simulink model "pfb_fir_generic_test_sim3"  (R2012b)
settings: Solver=VariableStepDiscrete  StartTime=0.0  StopTime=10.0  RelTol=1e-3
model workspace (MAT data in the model file):
  synci = [0 1 2 3 4 5 6 7 8 9 10 11 ... (589826 elements, 294913x2)]
  din0 = [0 1 2 3 4 5 6 7 8 9 10 11 ... (73730 elements, 36865x2)]
  din1 = [0 1 2 3 4 5 6 7 8 9 10 11 ... (73730 elements, 36865x2)]
  din2 = [0 1 2 3 4 5 6 7 8 9 10 11 ... (73730 elements, 36865x2)]
  din3 = [0 1 2 3 4 5 6 7 8 9 10 11 ... (73730 elements, 36865x2)]
  din4 = [0 1 2 3 4 5 6 7 8 9 10 11 ... (73730 elements, 36865x2)]
  din5 = [0 1 2 3 4 5 6 7 8 9 10 11 ... (73730 elements, 36865x2)]
  din6 = [0 1 2 3 4 5 6 7 8 9 10 11 ... (73730 elements, 36865x2)]
  din7 = [0 1 2 3 4 5 6 7 8 9 10 11 ... (73730 elements, 36865x2)]
libraries: xbsIndex_r4 x5585, casper_library_delays x1
(part 12 of 25)

== system pfb_fir_generic_test_sim3/pfb_fir_generic/pfb_fir_taps/bus_madd ==
  a : Inport
  b : Inport  Port=2
  c : Inport  Port=3
  en : Inport  Port=4
  Gateway Out{,1..23} (24 alike) : xbsIndex_r4/Gateway Out  inherit_from_input=off  hdl_port=on  timing_constraint=None  locs_specified=off  LOCs={}  UseAsDAC=off  DACChannel='1'  block_type=gatewayout
  To Workspace : ToWorkspace  VariableName=mult_ab_64  SampleTime=-1  SaveFormat=Timeseries
  To Workspace1 : ToWorkspace  VariableName=mult_ab_c_64  SampleTime=-1  SaveFormat=Timeseries
  To Workspace10 : ToWorkspace  VariableName=mult_a33  SampleTime=-1  SaveFormat=Structure With Time
  To Workspace11 : ToWorkspace  VariableName=mult_a32  SampleTime=-1  SaveFormat=Structure With Time
  To Workspace12 : ToWorkspace  VariableName=mult_a31  SampleTime=-1  SaveFormat=Structure With Time
  To Workspace13 : ToWorkspace  VariableName=mult_b33  SampleTime=-1  SaveFormat=Structure With Time
  To Workspace14 : ToWorkspace  VariableName=mult_b32  SampleTime=-1  SaveFormat=Structure With Time
  To Workspace15 : ToWorkspace  VariableName=mult_b31  SampleTime=-1  SaveFormat=Structure With Time
  To Workspace16 : ToWorkspace  VariableName=add_b_32  SampleTime=-1  SaveFormat=Structure With Time
  To Workspace17 : ToWorkspace  VariableName=add_b_33  SampleTime=-1  SaveFormat=Structure With Time
  To Workspace18 : ToWorkspace  VariableName=add_b_16  SampleTime=-1  SaveFormat=Structure With Time
  To Workspace19 : ToWorkspace  VariableName=add_b_48  SampleTime=-1  SaveFormat=Structure With Time
  To Workspace2 : ToWorkspace  VariableName=mult_ab_32  SampleTime=-1  SaveFormat=Structure With Time
  To Workspace20 : ToWorkspace  VariableName=add_b_17  SampleTime=-1  SaveFormat=Structure With Time
  To Workspace21 : ToWorkspace  VariableName=add_b_15  SampleTime=-1  SaveFormat=Structure With Time
  To Workspace22 : ToWorkspace  VariableName=add_b_47  SampleTime=-1  SaveFormat=Structure With Time
  To Workspace23 : ToWorkspace  VariableName=add_b_49  SampleTime=-1  SaveFormat=Structure With Time
  To Workspace3 : ToWorkspace  VariableName=mult_ab_c_33  SampleTime=-1  SaveFormat=Structure With Time
  To Workspace4 : ToWorkspace  VariableName=mult_ab_c_31  SampleTime=-1  SaveFormat=Structure With Time
  To Workspace5 : ToWorkspace  VariableName=mult_ab_33  SampleTime=-1  SaveFormat=Structure With Time
  To Workspace6 : ToWorkspace  VariableName=mult_ab_31  SampleTime=-1  SaveFormat=Structure With Time
  To Workspace7 : ToWorkspace  VariableName=mult_ab_c32  SampleTime=-1  SaveFormat=Structure With Time
  To Workspace8 : ToWorkspace  VariableName=mult_ab_c_34  SampleTime=-1  SaveFormat=Structure With Time
  To Workspace9 : ToWorkspace  VariableName=add_b_34  SampleTime=-1  SaveFormat=Structure With Time
  a*b+c_bussify : Subsystem  AncestorBlock=casper_library_flow_control/bus_create  mask(bus_create){inputNum=64}
      mask prompts: inputNum "Number of inputs:"
      mask init:
      | bus_create_init(gcb,...
      |     'inputNum', inputNum);
  a_debus : Subsystem  AncestorBlock=casper_library_flow_control/bus_expand  mask(bus_expand){mode=divisions of arbitrary size, outputNum=1, outputWidth=[10 10 10 10 10 10 10 10 10 10 10 10 10 10 10 10 10 10 10 10 10 10 10 10 10 10 10 10 10 10 10 10 10 10 10 10 10 10 10 10 10 10 10 10 10 10 10 10 10 10 10 10 10 10 10 10 10 10 10 10 10 10 10 10], outputBinaryPt=[9 9 9 9 9 9 9 9 9 9 9 9 9 9 9 9 9 9 9 9 9 9 9 9 9 9 9 9 9 9 9 9 9 9 9 9 9 9 9 9 9 9 9 9 9 9 9 9 9 9 9 9 9 9 9 9 9 9 9 9 9 9 9 9], outputArithmeticType=[1 1 1 1 1 1 1 1 1 1 1 1 1 1 1 1 1 1 1 1 1 1 1 1 1 1 1 1 1 1 1 1 1 1 1 1 1 1 1 1 1 1 1 1 1 1 1 1 1 1 1 1 1 1 1 1 1 1 1 1 1 1 1 1], show_format=on, outputToWorkspace=on, variablePrefix=mult_a, outputToModelAsWell=on}
      mask prompts: outputNum "Number of outputs:"; outputWidth "Output width [msb ... lsb]:"; outputBinaryPt "Output binary point position [msb ... lsb]:"; outputArithmeticType "Output arithmetic type (ufix=0, fix=1, bool=2) [msb ... lsb]:"; show_format "Print format string?"; outputToWorkspace "Output to workspace?"; variablePrefix "Variable name prefix:"; outputToModelAsWell "Output to model as well?"
      mask help:
      | Expands a 'bus' made using a bus_create or Xilinx
      | concat block.
      | The input will be divided into the specified number
      | of outputs with the specified arithmetic types.
      | Divisions are made from most significant bit.
      mask init: same as pfb_fir_generic_test_sim3/pfb_fir_generic/bus_expand
      settings: AttributesFormatString=64 outputs: f10.9,f10.9,f10.9,f10.9,f10.9,f10.9,f10.9,f10.9,f10.9,f10.9,f10.9,f10.9,f10.9,f10.9,f10.9,f10.9,f10.9,f10.9,f10.9,f10.9,f10.9,f10.9,f10.9,f10.9,f10.9,f10.9,f10.9,f10.9,f10.9,f10.9,f10.9,f10.9,f10.9,f10.9,f10.9,f10.9,f10.9,f10.9,f10.9,f10.9,f10.9,f10.9,f10.9,f10.9,f10.9,f10.9,f10.9,f10.9,f10.9,f10.9,f10.9,f10.9,f10.9,f10.9,f10.9,f10.9,f10.9,f10.9,f10.9,f10.9,f10.9,f10.9,f10.9,f10.9,, mult_a_?
      mask TypeOptions mode: divisions of equal size | divisions of arbitrary size
      mask Callback mode: bus_expand_callback();
      mask Callback outputWidth: bus_expand_callback();
      mask Callback outputToWorkspace: bus_expand_callback();
  addsub{1..16} (16 alike) : xbsIndex_r4/AddSub  mode=Addition  use_carryin=off  use_carryout=off  en=on  latency=1  precision=User Defined  arith_type="Signed  (2's comp)"  n_bits=28  bin_pt=26  quantization=Truncate  overflow=Wrap  dbl_ovrd=off  use_behavioral_HDL=on  hw_selection=Fabric  pipelined=on  block_type=addsub
  addsub{17..32} (16 alike) : xbsIndex_r4/AddSub  mode=Addition  use_carryin=off  use_carryout=off  en=on  latency=1  precision=User Defined  arith_type="Signed  (2's comp)"  n_bits=29  bin_pt=26  quantization=Truncate  overflow=Wrap  dbl_ovrd=off  use_behavioral_HDL=on  hw_selection=Fabric  pipelined=on  block_type=addsub
  addsub{33..48} (16 alike) : xbsIndex_r4/AddSub  mode=Addition  use_carryin=off  use_carryout=off  en=on  latency=1  precision=User Defined  arith_type="Signed  (2's comp)"  n_bits=30  bin_pt=26  quantization=Truncate  overflow=Wrap  dbl_ovrd=off  use_behavioral_HDL=on  hw_selection=Fabric  pipelined=on  block_type=addsub
  addsub{49..64} (16 alike) : xbsIndex_r4/AddSub  mode=Addition  use_carryin=off  use_carryout=off  en=on  latency=1  precision=User Defined  arith_type="Signed  (2's comp)"  n_bits=31  bin_pt=26  quantization=Truncate  overflow=Wrap  dbl_ovrd=off  use_behavioral_HDL=on  hw_selection=Fabric  pipelined=on  block_type=addsub
  b_debus : Subsystem  AncestorBlock=casper_library_flow_control/bus_expand  mask(bus_expand){mode=divisions of arbitrary size, outputNum=1, outputWidth=[18 18 18 18 18 18 18 18 18 18 18 18 18 18 18 18 18 18 18 18 18 18 18 18 18 18 18 18 18 18 18 18 18 18 18 18 18 18 18 18 18 18 18 18 18 18 18 18 18 18 18 18 18 18 18 18 18 18 18 18 18 18 18 18], outputBinaryPt=[17 17 17 17 17 17 17 17 17 17 17 17 17 17 17 17 17 17 17 17 17 17 17 17 17 17 17 17 17 17 17 17 17 17 17 17 17 17 17 17 17 17 17 17 17 17 17 17 17 17 17 17 17 17 17 17 17 17 17 17 17 17 17 17], outputArithmeticType=[1 1 1 1 1 1 1 1 1 1 1 1 1 1 1 1 1 1 1 1 1 1 1 1 1 1 1 1 1 1 1 1 1 1 1 1 1 1 1 1 1 1 1 1 1 1 1 1 1 1 1 1 1 1 1 1 1 1 1 1 1 1 1 1], show_format=on, outputToWorkspace=on, variablePrefix=mult_b, outputToModelAsWell=on}
      mask prompts: outputNum "Number of outputs:"; outputWidth "Output width [msb ... lsb]:"; outputBinaryPt "Output binary point position [msb ... lsb]:"; outputArithmeticType "Output arithmetic type (ufix=0, fix=1, bool=2) [msb ... lsb]:"; show_format "Print format string?"; outputToWorkspace "Output to workspace?"; variablePrefix "Variable name prefix:"; outputToModelAsWell "Output to model as well?"
      mask help:
      | Expands a 'bus' made using a bus_create or Xilinx
      | concat block.
      | The input will be divided into the specified number
      | of outputs with the specified arithmetic types.
      | Divisions are made from most significant bit.
      mask init: same as pfb_fir_generic_test_sim3/pfb_fir_generic/bus_expand
      settings: AttributesFormatString=64 outputs: f18.17,f18.17,f18.17,f18.17,f18.17,f18.17,f18.17,f18.17,f18.17,f18.17,f18.17,f18.17,f18.17,f18.17,f18.17,f18.17,f18.17,f18.17,f18.17,f18.17,f18.17,f18.17,f18.17,f18.17,f18.17,f18.17,f18.17,f18.17,f18.17,f18.17,f18.17,f18.17,f18.17,f18.17,f18.17,f18.17,f18.17,f18.17,f18.17,f18.17,f18.17,f18.17,f18.17,f18.17,f18.17,f18.17,f18.17,f18.17,f18.17,f18.17,f18.17,f18.17,f18.17,f18.17,f18.17,f18.17,f18.17,f18.17,f18.17,f18.17,f18.17,f18.17,f18.17,f18.17,, mult_b_?
      mask TypeOptions mode: divisions of equal size | divisions of arbitrary size
      mask Callback mode: bus_expand_callback();
      mask Callback outputWidth: bus_expand_callback();
      mask Callback outputToWorkspace: bus_expand_callback();
  c_debus : Subsystem  AncestorBlock=casper_library_flow_control/bus_expand  mask(bus_expand){mode=divisions of arbitrary size, outputNum=1, outputWidth=[28 28 28 28 28 28 28 28 28 28 28 28 28 28 28 28 28 28 28 28 28 28 28 28 28 28 28 28 28 28 28 28 29 29 29 29 29 29 29 29 29 29 29 29 29 29 29 29 30 30 30 30 30 30 30 30 30 30 30 30 30 30 30 30], outputBinaryPt=[26 26 26 26 26 26 26 26 26 26 26 26 26 26 26 26 26 26 26 26 26 26 26 26 26 26 26 26 26 26 26 26 26 26 26 26 26 26 26 26 26 26 26 26 26 26 26 26 26 26 26 26 26 26 26 26 26 26 26 26 26 26 26 26], outputArithmeticType=[1 1 1 1 1 1 1 1 1 1 1 1 1 1 1 1 1 1 1 1 1 1 1 1 1 1 1 1 1 1 1 1 1 1 1 1 1 1 1 1 1 1 1 1 1 1 1 1 1 1 1 1 1 1 1 1 1 1 1 1 1 1 1 1], show_format=on, outputToWorkspace=on, variablePrefix=add_c, outputToModelAsWell=on}
      mask prompts: outputNum "Number of outputs:"; outputWidth "Output width [msb ... lsb]:"; outputBinaryPt "Output binary point position [msb ... lsb]:"; outputArithmeticType "Output arithmetic type (ufix=0, fix=1, bool=2) [msb ... lsb]:"; show_format "Print format string?"; outputToWorkspace "Output to workspace?"; variablePrefix "Variable name prefix:"; outputToModelAsWell "Output to model as well?"
      mask help:
      | Expands a 'bus' made using a bus_create or Xilinx
      | concat block.
      | The input will be divided into the specified number
      | of outputs with the specified arithmetic types.
      | Divisions are made from most significant bit.
      mask init: same as pfb_fir_generic_test_sim3/pfb_fir_generic/bus_expand
      settings: AttributesFormatString=64 outputs: f28.26,f28.26,f28.26,f28.26,f28.26,f28.26,f28.26,f28.26,f28.26,f28.26,f28.26,f28.26,f28.26,f28.26,f28.26,f28.26,f28.26,f28.26,f28.26,f28.26,f28.26,f28.26,f28.26,f28.26,f28.26,f28.26,f28.26,f28.26,f28.26,f28.26,f28.26,f28.26,f29.26,f29.26,f29.26,f29.26,f29.26,f29.26,f29.26,f29.26,f29.26,f29.26,f29.26,f29.26,f29.26,f29.26,f29.26,f29.26,f30.26,f30.26,f30.26,f30.26,f30.26,f30.26,f30.26,f30.26,f30.26,f30.26,f30.26,f30.26,f30.26,f30.26,f30.26,f30.26,, add_c_?
      mask TypeOptions mode: divisions of equal size | divisions of arbitrary size
      mask Callback mode: bus_expand_callback();
      mask Callback outputWidth: bus_expand_callback();
      mask Callback outputToWorkspace: bus_expand_callback();
  den0 : xbsIndex_r4/Delay  rst=off  infoeditControl=Selection of Reset will increase slice count due to use of real FFs and instead of SRLs  en=off  latency=3  dbl_ovrd=off  reg_retiming=on  block_type=delay
  den1 : xbsIndex_r4/Delay  rst=off  infoeditControl=Selection of Reset will increase slice count due to use of real FFs and instead of SRLs  en=off  latency=1  dbl_ovrd=off  reg_retiming=on  block_type=delay
  den2 : xbsIndex_r4/Delay  rst=off  infoeditControl=Selection of Reset will increase slice count due to use of real FFs and instead of SRLs  en=off  latency=1  dbl_ovrd=off  reg_retiming=on  block_type=delay
  en_debus1 : Subsystem  AncestorBlock=casper_library_flow_control/bus_expand  mask(bus_expand){mode=divisions of equal size, outputNum=64, outputWidth=1, outputBinaryPt=0, outputArithmeticType=2, show_format=on, outputToWorkspace=on, variablePrefix=add_en, outputToModelAsWell=on}
      mask prompts: outputNum "Number of outputs:"; outputWidth "Output width:"; outputBinaryPt "Output binary point position:"; outputArithmeticType "Output arithmetic type (ufix=0, fix=1, bool=2):"; show_format "Print format string?"; outputToWorkspace "Output to workspace?"; variablePrefix "Variable name prefix:"; outputToModelAsWell "Output to model as well?"
      mask help:
      | Expands a 'bus' made using a bus_create or Xilinx
      | concat block.
      | The input will be divided into the specified number
      | of outputs with the specified arithmetic types.
      | Divisions are made from most significant bit.
      mask init: same as pfb_fir_generic_test_sim3/pfb_fir_generic/bus_expand
      settings: AttributesFormatString=64 outputs: b,b,b,b,b,b,b,b,b,b,b,b,b,b,b,b,b,b,b,b,b,b,b,b,b,b,b,b,b,b,b,b,b,b,b,b,b,b,b,b,b,b,b,b,b,b,b,b,b,b,b,b,b,b,b,b,b,b,b,b,b,b,b,b,, add_en_?
      mask TypeOptions mode: divisions of equal size | divisions of arbitrary size
      mask Callback mode: bus_expand_callback();
      mask Callback outputWidth: bus_expand_callback();
      mask Callback outputToWorkspace: bus_expand_callback();
  mult{1..64} (64 alike) : xbsIndex_r4/Mult  precision=Full  arith_type="Signed  (2's comp)"  n_bits=16  bin_pt=14  quantization=Truncate  overflow=Wrap  en=off  latency=3  dbl_ovrd=off  use_behavioral_HDL=on  opt=Speed  use_embedded=off  optimum_pipeline=off  pipeline=on  use_rpm=on  placement_style=Triangular  block_type=mult
  repa : Subsystem  AncestorBlock=casper_library_bus/bus_replicate  mask(bus_replicate){replication=1, latency=1, misc=off, implementation=core}
      mask prompts: replication "replication factor"; misc "misc support"; implementation "delay implementation"
      mask help: Output bus formed by replicating input bus a number of times
      mask init:
      | bus_replicate_init(gcb, ...
      |     'replication', replication, ...
      |     'latency', latency, ...
      |     'implementation', implementation, ...
      |     'misc', misc);
      mask TypeOptions implementation: core | behavioral
  repb : Subsystem  AncestorBlock=casper_library_bus/bus_replicate  mask(bus_replicate){replication=1, latency=1, misc=off, implementation=core}
      mask prompts: replication "replication factor"; misc "misc support"; implementation "delay implementation"
      mask help: Output bus formed by replicating input bus a number of times
      mask init:
      | bus_replicate_init(gcb, ...
      |     'replication', replication, ...
      |     'latency', latency, ...
      |     'implementation', implementation, ...
      |     'misc', misc);
      mask TypeOptions implementation: core | behavioral
  repen1 : Subsystem  AncestorBlock=casper_library_bus/bus_replicate  mask(bus_replicate){replication=64, latency=2, misc=off, implementation=core}
      mask prompts: replication "replication factor"; misc "misc support"; implementation "delay implementation"
      mask help: Output bus formed by replicating input bus a number of times
      mask init:
      | bus_replicate_init(gcb, ...
      |     'replication', replication, ...
      |     'latency', latency, ...
      |     'implementation', implementation, ...
      |     'misc', misc);
      mask TypeOptions implementation: core | behavioral
  a*b+c : Outport
  dvalid : Outport  Port=2
  wires:
  a/1 -> repa/1(in)
  b/1 -> repb/1(in)
  repa/1(out) -> a_debus/1(bus_in)
  repb/1(out) -> b_debus/1(bus_in)
  a_debus/1(msb_out64) -> mult1/1
  b_debus/1(msb_out64) -> mult1/2
  a_debus/2(out63) -> mult2/1
  b_debus/2(out63) -> mult2/2
  a_debus/3(out62) -> mult3/1
  b_debus/3(out62) -> mult3/2
  a_debus/4(out61) -> mult4/1
  b_debus/4(out61) -> mult4/2
  a_debus/5(out60) -> mult5/1
  b_debus/5(out60) -> mult5/2
  a_debus/6(out59) -> mult6/1
  b_debus/6(out59) -> mult6/2
  a_debus/7(out58) -> mult7/1
  b_debus/7(out58) -> mult7/2
  a_debus/8(out57) -> mult8/1
  b_debus/8(out57) -> mult8/2
  a_debus/9(out56) -> mult9/1
  b_debus/9(out56) -> mult9/2
  a_debus/10(out55) -> mult10/1
  b_debus/10(out55) -> mult10/2
  a_debus/11(out54) -> mult11/1
  b_debus/11(out54) -> mult11/2
  a_debus/12(out53) -> mult12/1
  b_debus/12(out53) -> mult12/2
  a_debus/13(out52) -> mult13/1
  b_debus/13(out52) -> mult13/2
  a_debus/14(out51) -> mult14/1
  b_debus/14(out51) -> mult14/2
  a_debus/15(out50) -> mult15/1
  b_debus/15(out50) -> mult15/2
  a_debus/16(out49) -> mult16/1
  b_debus/16(out49) -> mult16/2
  a_debus/17(out48) -> mult17/1
  b_debus/17(out48) -> mult17/2
  a_debus/18(out47) -> mult18/1
  b_debus/18(out47) -> mult18/2
  a_debus/19(out46) -> mult19/1
  b_debus/19(out46) -> mult19/2
  a_debus/20(out45) -> mult20/1
  b_debus/20(out45) -> mult20/2
  a_debus/21(out44) -> mult21/1
  b_debus/21(out44) -> mult21/2
  a_debus/22(out43) -> mult22/1
  b_debus/22(out43) -> mult22/2
  a_debus/23(out42) -> mult23/1
  b_debus/23(out42) -> mult23/2
  a_debus/24(out41) -> mult24/1
  b_debus/24(out41) -> mult24/2
  a_debus/25(out40) -> mult25/1
  b_debus/25(out40) -> mult25/2
  a_debus/26(out39) -> mult26/1
  b_debus/26(out39) -> mult26/2
  a_debus/27(out38) -> mult27/1
  b_debus/27(out38) -> mult27/2
  a_debus/28(out37) -> mult28/1
  b_debus/28(out37) -> mult28/2
  a_debus/29(out36) -> mult29/1
  b_debus/29(out36) -> mult29/2
  a_debus/30(out35) -> mult30/1
  b_debus/30(out35) -> mult30/2
  a_debus/31(out34) -> mult31/1
  b_debus/31(out34) -> mult31/2
  a_debus/32(out33) -> Gateway Out10/1, mult32/1
  b_debus/32(out33) -> Gateway Out13/1, mult32/2
  a_debus/33(out32) -> Gateway Out11/1, mult33/1
  b_debus/33(out32) -> Gateway Out14/1, mult33/2
  a_debus/34(out31) -> Gateway Out12/1, mult34/1
  b_debus/34(out31) -> Gateway Out15/1, mult34/2
  a_debus/35(out30) -> mult35/1
  b_debus/35(out30) -> mult35/2
  a_debus/36(out29) -> mult36/1
  b_debus/36(out29) -> mult36/2
  a_debus/37(out28) -> mult37/1
  b_debus/37(out28) -> mult37/2
  a_debus/38(out27) -> mult38/1
  b_debus/38(out27) -> mult38/2
  a_debus/39(out26) -> mult39/1
  b_debus/39(out26) -> mult39/2
  a_debus/40(out25) -> mult40/1
  b_debus/40(out25) -> mult40/2
  a_debus/41(out24) -> mult41/1
  b_debus/41(out24) -> mult41/2
  a_debus/42(out23) -> mult42/1
  b_debus/42(out23) -> mult42/2
  a_debus/43(out22) -> mult43/1
  b_debus/43(out22) -> mult43/2
  a_debus/44(out21) -> mult44/1
  b_debus/44(out21) -> mult44/2
  a_debus/45(out20) -> mult45/1
  b_debus/45(out20) -> mult45/2
  a_debus/46(out19) -> mult46/1
  b_debus/46(out19) -> mult46/2
  a_debus/47(out18) -> mult47/1
  b_debus/47(out18) -> mult47/2
  a_debus/48(out17) -> mult48/1
  b_debus/48(out17) -> mult48/2
  a_debus/49(out16) -> mult49/1
  b_debus/49(out16) -> mult49/2
  a_debus/50(out15) -> mult50/1
  b_debus/50(out15) -> mult50/2
  a_debus/51(out14) -> mult51/1
  b_debus/51(out14) -> mult51/2
  a_debus/52(out13) -> mult52/1
  b_debus/52(out13) -> mult52/2
  a_debus/53(out12) -> mult53/1
  b_debus/53(out12) -> mult53/2
  a_debus/54(out11) -> mult54/1
  b_debus/54(out11) -> mult54/2
  a_debus/55(out10) -> mult55/1
  b_debus/55(out10) -> mult55/2
  a_debus/56(out9) -> mult56/1
  b_debus/56(out9) -> mult56/2
  a_debus/57(out8) -> mult57/1
  b_debus/57(out8) -> mult57/2
  a_debus/58(out7) -> mult58/1
  b_debus/58(out7) -> mult58/2
  a_debus/59(out6) -> mult59/1
  b_debus/59(out6) -> mult59/2
  a_debus/60(out5) -> mult60/1
  b_debus/60(out5) -> mult60/2
  a_debus/61(out4) -> mult61/1
  b_debus/61(out4) -> mult61/2
  a_debus/62(out3) -> mult62/1
  b_debus/62(out3) -> mult62/2
  a_debus/63(out2) -> mult63/1
  b_debus/63(out2) -> mult63/2
  a_debus/64(lsb_out1) -> mult64/1
  b_debus/64(lsb_out1) -> mult64/2
  en/1 -> den0/1, repen1/1(in)
  den0/1 -> den1/1
  c/1 -> c_debus/1(bus_in)
  repen1/1(out) -> en_debus1/1(bus_in)
  mult1/1 -> Gateway Out/1, addsub1/1
  c_debus/1(msb_out64) -> addsub1/2
  en_debus1/1(msb_out64) -> addsub1/3
  mult2/1 -> addsub2/1
  c_debus/2(out63) -> addsub2/2
  en_debus1/2(out63) -> addsub2/3
  mult3/1 -> addsub3/1
  c_debus/3(out62) -> addsub3/2
  en_debus1/3(out62) -> addsub3/3
  mult4/1 -> addsub4/1
  c_debus/4(out61) -> addsub4/2
  en_debus1/4(out61) -> addsub4/3
  mult5/1 -> addsub5/1
  c_debus/5(out60) -> addsub5/2
  en_debus1/5(out60) -> addsub5/3
  mult6/1 -> addsub6/1
  c_debus/6(out59) -> addsub6/2
  en_debus1/6(out59) -> addsub6/3
  mult7/1 -> addsub7/1
  c_debus/7(out58) -> addsub7/2
  en_debus1/7(out58) -> addsub7/3
  mult8/1 -> addsub8/1
  c_debus/8(out57) -> addsub8/2
  en_debus1/8(out57) -> addsub8/3
  mult9/1 -> addsub9/1
  c_debus/9(out56) -> addsub9/2
  en_debus1/9(out56) -> addsub9/3
  mult10/1 -> addsub10/1
  c_debus/10(out55) -> addsub10/2
  en_debus1/10(out55) -> addsub10/3
  mult11/1 -> addsub11/1
  c_debus/11(out54) -> addsub11/2
  en_debus1/11(out54) -> addsub11/3
  mult12/1 -> addsub12/1
  c_debus/12(out53) -> addsub12/2
  en_debus1/12(out53) -> addsub12/3
  mult13/1 -> addsub13/1
  c_debus/13(out52) -> addsub13/2
  en_debus1/13(out52) -> addsub13/3
  mult14/1 -> addsub14/1
  c_debus/14(out51) -> addsub14/2
  en_debus1/14(out51) -> addsub14/3
  mult15/1 -> addsub15/1
  c_debus/15(out50) -> Gateway Out21/1, addsub15/2
  en_debus1/15(out50) -> addsub15/3
  mult16/1 -> addsub16/1
  c_debus/16(out49) -> Gateway Out18/1, addsub16/2
  en_debus1/16(out49) -> addsub16/3
  mult17/1 -> addsub17/1
  c_debus/17(out48) -> Gateway Out20/1, addsub17/2
  en_debus1/17(out48) -> addsub17/3
  mult18/1 -> addsub18/1
  c_debus/18(out47) -> addsub18/2
  en_debus1/18(out47) -> addsub18/3
  mult19/1 -> addsub19/1
  c_debus/19(out46) -> addsub19/2
  en_debus1/19(out46) -> addsub19/3
  mult20/1 -> addsub20/1
  c_debus/20(out45) -> addsub20/2
  en_debus1/20(out45) -> addsub20/3
  mult21/1 -> addsub21/1
  c_debus/21(out44) -> addsub21/2
  en_debus1/21(out44) -> addsub21/3
  mult22/1 -> addsub22/1
  c_debus/22(out43) -> addsub22/2
  en_debus1/22(out43) -> addsub22/3
  mult23/1 -> addsub23/1
  c_debus/23(out42) -> addsub23/2
  en_debus1/23(out42) -> addsub23/3
  mult24/1 -> addsub24/1
  c_debus/24(out41) -> addsub24/2
  en_debus1/24(out41) -> addsub24/3
  mult25/1 -> addsub25/1
  c_debus/25(out40) -> addsub25/2
  en_debus1/25(out40) -> addsub25/3
  mult26/1 -> addsub26/1
  c_debus/26(out39) -> addsub26/2
  en_debus1/26(out39) -> addsub26/3
  mult27/1 -> addsub27/1
  c_debus/27(out38) -> addsub27/2
  en_debus1/27(out38) -> addsub27/3
  mult28/1 -> addsub28/1
  c_debus/28(out37) -> addsub28/2
  en_debus1/28(out37) -> addsub28/3
  mult29/1 -> addsub29/1
  c_debus/29(out36) -> addsub29/2
  en_debus1/29(out36) -> addsub29/3
  mult30/1 -> addsub30/1
  c_debus/30(out35) -> addsub30/2
  en_debus1/30(out35) -> addsub30/3
  mult31/1 -> addsub31/1
  c_debus/31(out34) -> addsub31/2
  en_debus1/31(out34) -> addsub31/3
  mult32/1 -> Gateway Out5/1, addsub32/1
  c_debus/32(out33) -> Gateway Out16/1, addsub32/2
  en_debus1/32(out33) -> addsub32/3
  mult33/1 -> Gateway Out2/1, addsub33/1
  en_debus1/33(out32) -> addsub33/3
  mult34/1 -> Gateway Out6/1, addsub34/1
  c_debus/34(out31) -> Gateway Out17/1, addsub34/2
  en_debus1/34(out31) -> addsub34/3
  mult35/1 -> addsub35/1
  c_debus/35(out30) -> addsub35/2
  en_debus1/35(out30) -> addsub35/3
  mult36/1 -> addsub36/1
  c_debus/36(out29) -> addsub36/2
  en_debus1/36(out29) -> addsub36/3
  mult37/1 -> addsub37/1
  c_debus/37(out28) -> addsub37/2
  en_debus1/37(out28) -> addsub37/3
  mult38/1 -> addsub38/1
  c_debus/38(out27) -> addsub38/2
  en_debus1/38(out27) -> addsub38/3
  mult39/1 -> addsub39/1
  c_debus/39(out26) -> addsub39/2
  en_debus1/39(out26) -> addsub39/3
  mult40/1 -> addsub40/1
  c_debus/40(out25) -> addsub40/2
  en_debus1/40(out25) -> addsub40/3
  mult41/1 -> addsub41/1
  c_debus/41(out24) -> addsub41/2
  en_debus1/41(out24) -> addsub41/3
  mult42/1 -> addsub42/1
  c_debus/42(out23) -> addsub42/2
  en_debus1/42(out23) -> addsub42/3
  mult43/1 -> addsub43/1
  c_debus/43(out22) -> addsub43/2
  en_debus1/43(out22) -> addsub43/3
  mult44/1 -> addsub44/1
  c_debus/44(out21) -> addsub44/2
  en_debus1/44(out21) -> addsub44/3
  mult45/1 -> addsub45/1
  c_debus/45(out20) -> addsub45/2
  en_debus1/45(out20) -> addsub45/3
  mult46/1 -> addsub46/1
  c_debus/46(out19) -> addsub46/2
  en_debus1/46(out19) -> addsub46/3
  mult47/1 -> addsub47/1
  c_debus/47(out18) -> Gateway Out22/1, addsub47/2
  en_debus1/47(out18) -> addsub47/3
  mult48/1 -> addsub48/1
  c_debus/48(out17) -> Gateway Out19/1, addsub48/2
  en_debus1/48(out17) -> addsub48/3
  mult49/1 -> addsub49/1
  c_debus/49(out16) -> Gateway Out23/1, addsub49/2
  en_debus1/49(out16) -> addsub49/3
  mult50/1 -> addsub50/1
  c_debus/50(out15) -> addsub50/2
  en_debus1/50(out15) -> addsub50/3
  mult51/1 -> addsub51/1
  c_debus/51(out14) -> addsub51/2
  en_debus1/51(out14) -> addsub51/3
  mult52/1 -> addsub52/1
  c_debus/52(out13) -> addsub52/2
  en_debus1/52(out13) -> addsub52/3
  mult53/1 -> addsub53/1
  c_debus/53(out12) -> addsub53/2
  en_debus1/53(out12) -> addsub53/3
  mult54/1 -> addsub54/1
  c_debus/54(out11) -> addsub54/2
  en_debus1/54(out11) -> addsub54/3
  mult55/1 -> addsub55/1
  c_debus/55(out10) -> addsub55/2
  en_debus1/55(out10) -> addsub55/3
  mult56/1 -> addsub56/1
  c_debus/56(out9) -> addsub56/2
  en_debus1/56(out9) -> addsub56/3
  mult57/1 -> addsub57/1
  c_debus/57(out8) -> addsub57/2
  en_debus1/57(out8) -> addsub57/3
  mult58/1 -> addsub58/1
  c_debus/58(out7) -> addsub58/2
  en_debus1/58(out7) -> addsub58/3
  mult59/1 -> addsub59/1
  c_debus/59(out6) -> addsub59/2
  en_debus1/59(out6) -> addsub59/3
  mult60/1 -> addsub60/1
  c_debus/60(out5) -> addsub60/2
  en_debus1/60(out5) -> addsub60/3
  mult61/1 -> addsub61/1
  c_debus/61(out4) -> addsub61/2
  en_debus1/61(out4) -> addsub61/3
  mult62/1 -> addsub62/1
  c_debus/62(out3) -> addsub62/2
  en_debus1/62(out3) -> addsub62/3
  mult63/1 -> addsub63/1
  c_debus/63(out2) -> addsub63/2
  en_debus1/63(out2) -> addsub63/3
  mult64/1 -> addsub64/1
  c_debus/64(lsb_out1) -> addsub64/2
  en_debus1/64(lsb_out1) -> addsub64/3
  den1/1 -> den2/1
  addsub1/1 -> Gateway Out1/1, a*b+c_bussify/1(in1)
  addsub2/1 -> a*b+c_bussify/2(in2)
  addsub3/1 -> a*b+c_bussify/3(in3)
  addsub4/1 -> a*b+c_bussify/4(in4)
  addsub5/1 -> a*b+c_bussify/5(in5)
  addsub6/1 -> a*b+c_bussify/6(in6)
  addsub7/1 -> a*b+c_bussify/7(in7)
  addsub8/1 -> a*b+c_bussify/8(in8)
  addsub9/1 -> a*b+c_bussify/9(in9)
  addsub10/1 -> a*b+c_bussify/10(in10)
  addsub11/1 -> a*b+c_bussify/11(in11)
  addsub12/1 -> a*b+c_bussify/12(in12)
  addsub13/1 -> a*b+c_bussify/13(in13)
  addsub14/1 -> a*b+c_bussify/14(in14)
  addsub15/1 -> a*b+c_bussify/15(in15)
  addsub16/1 -> a*b+c_bussify/16(in16)
  addsub17/1 -> a*b+c_bussify/17(in17)
  addsub18/1 -> a*b+c_bussify/18(in18)
  addsub19/1 -> a*b+c_bussify/19(in19)
  addsub20/1 -> a*b+c_bussify/20(in20)
  addsub21/1 -> a*b+c_bussify/21(in21)
  addsub22/1 -> a*b+c_bussify/22(in22)
  addsub23/1 -> a*b+c_bussify/23(in23)
  addsub24/1 -> a*b+c_bussify/24(in24)
  addsub25/1 -> a*b+c_bussify/25(in25)
  addsub26/1 -> a*b+c_bussify/26(in26)
  addsub27/1 -> a*b+c_bussify/27(in27)
  addsub28/1 -> a*b+c_bussify/28(in28)
  addsub29/1 -> a*b+c_bussify/29(in29)
  addsub30/1 -> a*b+c_bussify/30(in30)
  addsub31/1 -> Gateway Out4/1, a*b+c_bussify/31(in31)
  addsub32/1 -> Gateway Out7/1, a*b+c_bussify/32(in32)
  addsub33/1 -> Gateway Out3/1, a*b+c_bussify/33(in33)
  addsub34/1 -> Gateway Out8/1, a*b+c_bussify/34(in34)
  addsub35/1 -> a*b+c_bussify/35(in35)
  addsub36/1 -> a*b+c_bussify/36(in36)
  addsub37/1 -> a*b+c_bussify/37(in37)
  addsub38/1 -> a*b+c_bussify/38(in38)
  addsub39/1 -> a*b+c_bussify/39(in39)
  addsub40/1 -> a*b+c_bussify/40(in40)
  addsub41/1 -> a*b+c_bussify/41(in41)
  addsub42/1 -> a*b+c_bussify/42(in42)
  addsub43/1 -> a*b+c_bussify/43(in43)
  addsub44/1 -> a*b+c_bussify/44(in44)
  addsub45/1 -> a*b+c_bussify/45(in45)
  addsub46/1 -> a*b+c_bussify/46(in46)
  addsub47/1 -> a*b+c_bussify/47(in47)
  addsub48/1 -> a*b+c_bussify/48(in48)
  addsub49/1 -> a*b+c_bussify/49(in49)
  addsub50/1 -> a*b+c_bussify/50(in50)
  addsub51/1 -> a*b+c_bussify/51(in51)
  addsub52/1 -> a*b+c_bussify/52(in52)
  addsub53/1 -> a*b+c_bussify/53(in53)
  addsub54/1 -> a*b+c_bussify/54(in54)
  addsub55/1 -> a*b+c_bussify/55(in55)
  addsub56/1 -> a*b+c_bussify/56(in56)
  addsub57/1 -> a*b+c_bussify/57(in57)
  addsub58/1 -> a*b+c_bussify/58(in58)
  addsub59/1 -> a*b+c_bussify/59(in59)
  addsub60/1 -> a*b+c_bussify/60(in60)
  addsub61/1 -> a*b+c_bussify/61(in61)
  addsub62/1 -> a*b+c_bussify/62(in62)
  addsub63/1 -> a*b+c_bussify/63(in63)
  addsub64/1 -> a*b+c_bussify/64(in64)
  a*b+c_bussify/1(bus_out) -> a*b+c/1
  den2/1 -> dvalid/1
  Gateway Out/1 -> To Workspace/1
  Gateway Out1/1 -> To Workspace1/1
  Gateway Out2/1 -> To Workspace2/1
  Gateway Out3/1 -> To Workspace3/1
  Gateway Out4/1 -> To Workspace4/1
  Gateway Out5/1 -> To Workspace5/1
  Gateway Out6/1 -> To Workspace6/1
  Gateway Out7/1 -> To Workspace7/1
  Gateway Out8/1 -> To Workspace8/1
  Gateway Out9/1 -> To Workspace17/1
  c_debus/33(out32) -> Gateway Out9/1, addsub33/2
  Gateway Out10/1 -> To Workspace10/1
  Gateway Out11/1 -> To Workspace11/1
  Gateway Out12/1 -> To Workspace12/1
  Gateway Out13/1 -> To Workspace13/1
  Gateway Out14/1 -> To Workspace14/1
  Gateway Out15/1 -> To Workspace15/1
  Gateway Out16/1 -> To Workspace16/1
  Gateway Out17/1 -> To Workspace9/1
  Gateway Out18/1 -> To Workspace18/1
  Gateway Out19/1 -> To Workspace19/1
  Gateway Out20/1 -> To Workspace20/1
  Gateway Out21/1 -> To Workspace21/1
  Gateway Out22/1 -> To Workspace22/1
  Gateway Out23/1 -> To Workspace23/1

== system pfb_fir_generic_test_sim3/pfb_fir_generic/pfb_fir_taps/ddata0 ==
  din : Inport
  en : Inport  Port=2
  del{1..32} (32 alike) : xbsIndex_r4/Delay  rst=off  infoeditControl=Selection of Reset will increase slice count due to use of real FFs and instead of SRLs  en=on  latency=2  dbl_ovrd=off  reg_retiming=on  block_type=delay
  din_expand : Subsystem  AncestorBlock=casper_library_flow_control/bus_expand  mask(bus_expand){mode=divisions of arbitrary size, outputNum=1, outputWidth=[10  10  10  10  10  10  10  10  10  10  10  10  10  10  10  10  10  10  10  10  10  10  10  10  10  10  10  10  10  10  10  10], outputBinaryPt=[0  0  0  0  0  0  0  0  0  0  0  0  0  0  0  0  0  0  0  0  0  0  0  0  0  0  0  0  0  0  0  0], outputArithmeticType=[0  0  0  0  0  0  0  0  0  0  0  0  0  0  0  0  0  0  0  0  0  0  0  0  0  0  0  0  0  0  0  0], show_format=on, outputToWorkspace=off, variablePrefix=, outputToModelAsWell=on}
      mask prompts: outputNum "Number of outputs:"; outputWidth "Output width [msb ... lsb]:"; outputBinaryPt "Output binary point position [msb ... lsb]:"; outputArithmeticType "Output arithmetic type (ufix=0, fix=1, bool=2) [msb ... lsb]:"; show_format "Print format string?"; outputToWorkspace "Output to workspace?"; variablePrefix "Variable name prefix:"; outputToModelAsWell "Output to model as well?"
      mask help:
      | Expands a 'bus' made using a bus_create or Xilinx
      | concat block.
      | The input will be divided into the specified number
      | of outputs with the specified arithmetic types.
      | Divisions are made from most significant bit.
      mask init: same as pfb_fir_generic_test_sim3/pfb_fir_generic/bus_expand
      settings: AttributesFormatString=32 outputs: uf10.0,uf10.0,uf10.0,uf10.0,uf10.0,uf10.0,uf10.0,uf10.0,uf10.0,uf10.0,uf10.0,uf10.0,uf10.0,uf10.0,uf10.0,uf10.0,uf10.0,uf10.0,uf10.0,uf10.0,uf10.0,uf10.0,uf10.0,uf10.0,uf10.0,uf10.0,uf10.0,uf10.0,uf10.0,uf10.0,uf10.0,uf10.0,
      mask TypeOptions mode: divisions of equal size | divisions of arbitrary size
      mask Callback mode: bus_expand_callback();
      mask Callback outputWidth: bus_expand_callback();
      mask Callback outputToWorkspace: bus_expand_callback();
  dout_compress : Subsystem  AncestorBlock=casper_library_flow_control/bus_create  mask(bus_create){inputNum=32}
      mask prompts: inputNum "Number of inputs:"
      mask init:
      | bus_create_init(gcb,...
      |     'inputNum', inputNum);
  en_expand : Subsystem  AncestorBlock=casper_library_flow_control/bus_expand  mask(bus_expand){mode=divisions of equal size, outputNum=32, outputWidth=1, outputBinaryPt=0, outputArithmeticType=2, show_format=on, outputToWorkspace=off, variablePrefix=, outputToModelAsWell=on}
      mask prompts: outputNum "Number of outputs:"; outputWidth "Output width:"; outputBinaryPt "Output binary point position:"; outputArithmeticType "Output arithmetic type (ufix=0, fix=1, bool=2):"; show_format "Print format string?"; outputToWorkspace "Output to workspace?"; variablePrefix "Variable name prefix:"; outputToModelAsWell "Output to model as well?"
      mask help:
      | Expands a 'bus' made using a bus_create or Xilinx
      | concat block.
      | The input will be divided into the specified number
      | of outputs with the specified arithmetic types.
      | Divisions are made from most significant bit.
      mask init: same as pfb_fir_generic_test_sim3/pfb_fir_generic/bus_expand
      settings: AttributesFormatString=32 outputs: b,b,b,b,b,b,b,b,b,b,b,b,b,b,b,b,b,b,b,b,b,b,b,b,b,b,b,b,b,b,b,b,
      mask TypeOptions mode: divisions of equal size | divisions of arbitrary size
      mask Callback mode: bus_expand_callback();
      mask Callback outputWidth: bus_expand_callback();
      mask Callback outputToWorkspace: bus_expand_callback();
  dout : Outport
  wires:
  din/1 -> din_expand/1(bus_in)
  en/1 -> en_expand/1(bus_in)
  din_expand/1(msb_out32) -> del1/1
  en_expand/1(msb_out32) -> del1/2
  din_expand/2(out31) -> del2/1
  en_expand/2(out31) -> del2/2
  din_expand/3(out30) -> del3/1
  en_expand/3(out30) -> del3/2
  din_expand/4(out29) -> del4/1
  en_expand/4(out29) -> del4/2
  din_expand/5(out28) -> del5/1
  en_expand/5(out28) -> del5/2
  din_expand/6(out27) -> del6/1
  en_expand/6(out27) -> del6/2
  din_expand/7(out26) -> del7/1
  en_expand/7(out26) -> del7/2
  din_expand/8(out25) -> del8/1
  en_expand/8(out25) -> del8/2
  din_expand/9(out24) -> del9/1
  en_expand/9(out24) -> del9/2
  din_expand/10(out23) -> del10/1
  en_expand/10(out23) -> del10/2
  din_expand/11(out22) -> del11/1
  en_expand/11(out22) -> del11/2
  din_expand/12(out21) -> del12/1
  en_expand/12(out21) -> del12/2
  din_expand/13(out20) -> del13/1
  en_expand/13(out20) -> del13/2
  din_expand/14(out19) -> del14/1
  en_expand/14(out19) -> del14/2
  din_expand/15(out18) -> del15/1
  en_expand/15(out18) -> del15/2
  din_expand/16(out17) -> del16/1
  en_expand/16(out17) -> del16/2
  din_expand/17(out16) -> del17/1
  en_expand/17(out16) -> del17/2
  din_expand/18(out15) -> del18/1
  en_expand/18(out15) -> del18/2
  din_expand/19(out14) -> del19/1
  en_expand/19(out14) -> del19/2
  din_expand/20(out13) -> del20/1
  en_expand/20(out13) -> del20/2
  din_expand/21(out12) -> del21/1
  en_expand/21(out12) -> del21/2
  din_expand/22(out11) -> del22/1
  en_expand/22(out11) -> del22/2
  din_expand/23(out10) -> del23/1
  en_expand/23(out10) -> del23/2
  din_expand/24(out9) -> del24/1
  en_expand/24(out9) -> del24/2
  din_expand/25(out8) -> del25/1
  en_expand/25(out8) -> del25/2
  din_expand/26(out7) -> del26/1
  en_expand/26(out7) -> del26/2
  din_expand/27(out6) -> del27/1
  en_expand/27(out6) -> del27/2
  din_expand/28(out5) -> del28/1
  en_expand/28(out5) -> del28/2
  din_expand/29(out4) -> del29/1
  en_expand/29(out4) -> del29/2
  din_expand/30(out3) -> del30/1
  en_expand/30(out3) -> del30/2
  din_expand/31(out2) -> del31/1
  en_expand/31(out2) -> del31/2
  din_expand/32(lsb_out1) -> del32/1
  en_expand/32(lsb_out1) -> del32/2
  del1/1 -> dout_compress/1(in1)
  del2/1 -> dout_compress/2(in2)
  del3/1 -> dout_compress/3(in3)
  del4/1 -> dout_compress/4(in4)
  del5/1 -> dout_compress/5(in5)
  del6/1 -> dout_compress/6(in6)
  del7/1 -> dout_compress/7(in7)
  del8/1 -> dout_compress/8(in8)
  del9/1 -> dout_compress/9(in9)
  del10/1 -> dout_compress/10(in10)
  del11/1 -> dout_compress/11(in11)
  del12/1 -> dout_compress/12(in12)
  del13/1 -> dout_compress/13(in13)
  del14/1 -> dout_compress/14(in14)
  del15/1 -> dout_compress/15(in15)
  del16/1 -> dout_compress/16(in16)
  del17/1 -> dout_compress/17(in17)
  del18/1 -> dout_compress/18(in18)
  del19/1 -> dout_compress/19(in19)
  del20/1 -> dout_compress/20(in20)
  del21/1 -> dout_compress/21(in21)
  del22/1 -> dout_compress/22(in22)
  del23/1 -> dout_compress/23(in23)
  del24/1 -> dout_compress/24(in24)
  del25/1 -> dout_compress/25(in25)
  del26/1 -> dout_compress/26(in26)
  del27/1 -> dout_compress/27(in27)
  del28/1 -> dout_compress/28(in28)
  del29/1 -> dout_compress/29(in29)
  del30/1 -> dout_compress/30(in30)
  del31/1 -> dout_compress/31(in31)
  del32/1 -> dout_compress/32(in32)
  dout_compress/1(bus_out) -> dout/1

== system pfb_fir_generic_test_sim3/pfb_fir_generic/pfb_fir_taps/ddata1 ==
  din : Inport
  en : Inport  Port=2
  del{1..48} (48 alike) : xbsIndex_r4/Delay  rst=off  infoeditControl=Selection of Reset will increase slice count due to use of real FFs and instead of SRLs  en=on  latency=2  dbl_ovrd=off  reg_retiming=on  block_type=delay
  din_expand : Subsystem  AncestorBlock=casper_library_flow_control/bus_expand  mask(bus_expand){mode=divisions of arbitrary size, outputNum=1, outputWidth=[10  10  10  10  10  10  10  10  10  10  10  10  10  10  10  10  10  10  10  10  10  10  10  10  10  10  10  10  10  10  10  10  10  10  10  10  10  10  10  10  10  10  10  10  10  10  10  10], outputBinaryPt=[0  0  0  0  0  0  0  0  0  0  0  0  0  0  0  0  0  0  0  0  0  0  0  0  0  0  0  0  0  0  0  0  0  0  0  0  0  0  0  0  0  0  0  0  0  0  0  0], outputArithmeticType=[0  0  0  0  0  0  0  0  0  0  0  0  0  0  0  0  0  0  0  0  0  0  0  0  0  0  0  0  0  0  0  0  0  0  0  0  0  0  0  0  0  0  0  0  0  0  0  0], show_format=on, outputToWorkspace=off, variablePrefix=, outputToModelAsWell=on}
      mask prompts: outputNum "Number of outputs:"; outputWidth "Output width [msb ... lsb]:"; outputBinaryPt "Output binary point position [msb ... lsb]:"; outputArithmeticType "Output arithmetic type (ufix=0, fix=1, bool=2) [msb ... lsb]:"; show_format "Print format string?"; outputToWorkspace "Output to workspace?"; variablePrefix "Variable name prefix:"; outputToModelAsWell "Output to model as well?"
      mask help:
      | Expands a 'bus' made using a bus_create or Xilinx
      | concat block.
      | The input will be divided into the specified number
      | of outputs with the specified arithmetic types.
      | Divisions are made from most significant bit.
      mask init: same as pfb_fir_generic_test_sim3/pfb_fir_generic/bus_expand
      settings: AttributesFormatString=48 outputs: uf10.0,uf10.0,uf10.0,uf10.0,uf10.0,uf10.0,uf10.0,uf10.0,uf10.0,uf10.0,uf10.0,uf10.0,uf10.0,uf10.0,uf10.0,uf10.0,uf10.0,uf10.0,uf10.0,uf10.0,uf10.0,uf10.0,uf10.0,uf10.0,uf10.0,uf10.0,uf10.0,uf10.0,uf10.0,uf10.0,uf10.0,uf10.0,uf10.0,uf10.0,uf10.0,uf10.0,uf10.0,uf10.0,uf10.0,uf10.0,uf10.0,uf10.0,uf10.0,uf10.0,uf10.0,uf10.0,uf10.0,uf10.0,
      mask TypeOptions mode: divisions of equal size | divisions of arbitrary size
      mask Callback mode: bus_expand_callback();
      mask Callback outputWidth: bus_expand_callback();
      mask Callback outputToWorkspace: bus_expand_callback();
  dout_compress : Subsystem  AncestorBlock=casper_library_flow_control/bus_create  mask(bus_create){inputNum=48}
      mask prompts: inputNum "Number of inputs:"
      mask init:
      | bus_create_init(gcb,...
      |     'inputNum', inputNum);
  en_expand : Subsystem  AncestorBlock=casper_library_flow_control/bus_expand  mask(bus_expand){mode=divisions of equal size, outputNum=48, outputWidth=1, outputBinaryPt=0, outputArithmeticType=2, show_format=on, outputToWorkspace=off, variablePrefix=, outputToModelAsWell=on}
      mask prompts: outputNum "Number of outputs:"; outputWidth "Output width:"; outputBinaryPt "Output binary point position:"; outputArithmeticType "Output arithmetic type (ufix=0, fix=1, bool=2):"; show_format "Print format string?"; outputToWorkspace "Output to workspace?"; variablePrefix "Variable name prefix:"; outputToModelAsWell "Output to model as well?"
      mask help:
      | Expands a 'bus' made using a bus_create or Xilinx
      | concat block.
      | The input will be divided into the specified number
      | of outputs with the specified arithmetic types.
      | Divisions are made from most significant bit.
      mask init: same as pfb_fir_generic_test_sim3/pfb_fir_generic/bus_expand
      settings: AttributesFormatString=48 outputs: b,b,b,b,b,b,b,b,b,b,b,b,b,b,b,b,b,b,b,b,b,b,b,b,b,b,b,b,b,b,b,b,b,b,b,b,b,b,b,b,b,b,b,b,b,b,b,b,
      mask TypeOptions mode: divisions of equal size | divisions of arbitrary size
      mask Callback mode: bus_expand_callback();
      mask Callback outputWidth: bus_expand_callback();
      mask Callback outputToWorkspace: bus_expand_callback();
  dout : Outport
  wires:
  din/1 -> din_expand/1(bus_in)
  en/1 -> en_expand/1(bus_in)
  din_expand/1(msb_out48) -> del1/1
  en_expand/1(msb_out48) -> del1/2
  din_expand/2(out47) -> del2/1
  en_expand/2(out47) -> del2/2
  din_expand/3(out46) -> del3/1
  en_expand/3(out46) -> del3/2
  din_expand/4(out45) -> del4/1
  en_expand/4(out45) -> del4/2
  din_expand/5(out44) -> del5/1
  en_expand/5(out44) -> del5/2
  din_expand/6(out43) -> del6/1
  en_expand/6(out43) -> del6/2
  din_expand/7(out42) -> del7/1
  en_expand/7(out42) -> del7/2
  din_expand/8(out41) -> del8/1
  en_expand/8(out41) -> del8/2
  din_expand/9(out40) -> del9/1
  en_expand/9(out40) -> del9/2
  din_expand/10(out39) -> del10/1
  en_expand/10(out39) -> del10/2
  din_expand/11(out38) -> del11/1
  en_expand/11(out38) -> del11/2
  din_expand/12(out37) -> del12/1
  en_expand/12(out37) -> del12/2
  din_expand/13(out36) -> del13/1
  en_expand/13(out36) -> del13/2
  din_expand/14(out35) -> del14/1
  en_expand/14(out35) -> del14/2
  din_expand/15(out34) -> del15/1
  en_expand/15(out34) -> del15/2
  din_expand/16(out33) -> del16/1
  en_expand/16(out33) -> del16/2
  din_expand/17(out32) -> del17/1
  en_expand/17(out32) -> del17/2
  din_expand/18(out31) -> del18/1
  en_expand/18(out31) -> del18/2
  din_expand/19(out30) -> del19/1
  en_expand/19(out30) -> del19/2
  din_expand/20(out29) -> del20/1
  en_expand/20(out29) -> del20/2
  din_expand/21(out28) -> del21/1
  en_expand/21(out28) -> del21/2
  din_expand/22(out27) -> del22/1
  en_expand/22(out27) -> del22/2
  din_expand/23(out26) -> del23/1
  en_expand/23(out26) -> del23/2
  din_expand/24(out25) -> del24/1
  en_expand/24(out25) -> del24/2
  din_expand/25(out24) -> del25/1
  en_expand/25(out24) -> del25/2
  din_expand/26(out23) -> del26/1
  en_expand/26(out23) -> del26/2
  din_expand/27(out22) -> del27/1
  en_expand/27(out22) -> del27/2
  din_expand/28(out21) -> del28/1
  en_expand/28(out21) -> del28/2
  din_expand/29(out20) -> del29/1
  en_expand/29(out20) -> del29/2
  din_expand/30(out19) -> del30/1
  en_expand/30(out19) -> del30/2
  din_expand/31(out18) -> del31/1
  en_expand/31(out18) -> del31/2
  din_expand/32(out17) -> del32/1
  en_expand/32(out17) -> del32/2
  din_expand/33(out16) -> del33/1
  en_expand/33(out16) -> del33/2
  din_expand/34(out15) -> del34/1
  en_expand/34(out15) -> del34/2
  din_expand/35(out14) -> del35/1
  en_expand/35(out14) -> del35/2
  din_expand/36(out13) -> del36/1
  en_expand/36(out13) -> del36/2
  din_expand/37(out12) -> del37/1
  en_expand/37(out12) -> del37/2
  din_expand/38(out11) -> del38/1
  en_expand/38(out11) -> del38/2
  din_expand/39(out10) -> del39/1
  en_expand/39(out10) -> del39/2
  din_expand/40(out9) -> del40/1
  en_expand/40(out9) -> del40/2
  din_expand/41(out8) -> del41/1
  en_expand/41(out8) -> del41/2
  din_expand/42(out7) -> del42/1
  en_expand/42(out7) -> del42/2
  din_expand/43(out6) -> del43/1
  en_expand/43(out6) -> del43/2
  din_expand/44(out5) -> del44/1
  en_expand/44(out5) -> del44/2
  din_expand/45(out4) -> del45/1
  en_expand/45(out4) -> del45/2
  din_expand/46(out3) -> del46/1
  en_expand/46(out3) -> del46/2
  din_expand/47(out2) -> del47/1
  en_expand/47(out2) -> del47/2
  din_expand/48(lsb_out1) -> del48/1
  en_expand/48(lsb_out1) -> del48/2
  del1/1 -> dout_compress/1(in1)
  del2/1 -> dout_compress/2(in2)
  del3/1 -> dout_compress/3(in3)
  del4/1 -> dout_compress/4(in4)
  del5/1 -> dout_compress/5(in5)
  del6/1 -> dout_compress/6(in6)
  del7/1 -> dout_compress/7(in7)
  del8/1 -> dout_compress/8(in8)
  del9/1 -> dout_compress/9(in9)
  del10/1 -> dout_compress/10(in10)
  del11/1 -> dout_compress/11(in11)
  del12/1 -> dout_compress/12(in12)
  del13/1 -> dout_compress/13(in13)
  del14/1 -> dout_compress/14(in14)
  del15/1 -> dout_compress/15(in15)
  del16/1 -> dout_compress/16(in16)
  del17/1 -> dout_compress/17(in17)
  del18/1 -> dout_compress/18(in18)
  del19/1 -> dout_compress/19(in19)
  del20/1 -> dout_compress/20(in20)
  del21/1 -> dout_compress/21(in21)
  del22/1 -> dout_compress/22(in22)
  del23/1 -> dout_compress/23(in23)
  del24/1 -> dout_compress/24(in24)
  del25/1 -> dout_compress/25(in25)
  del26/1 -> dout_compress/26(in26)
  del27/1 -> dout_compress/27(in27)
  del28/1 -> dout_compress/28(in28)
  del29/1 -> dout_compress/29(in29)
  del30/1 -> dout_compress/30(in30)
  del31/1 -> dout_compress/31(in31)
  del32/1 -> dout_compress/32(in32)
  del33/1 -> dout_compress/33(in33)
  del34/1 -> dout_compress/34(in34)
  del35/1 -> dout_compress/35(in35)
  del36/1 -> dout_compress/36(in36)
  del37/1 -> dout_compress/37(in37)
  del38/1 -> dout_compress/38(in38)
  del39/1 -> dout_compress/39(in39)
  del40/1 -> dout_compress/40(in40)
  del41/1 -> dout_compress/41(in41)
  del42/1 -> dout_compress/42(in42)
  del43/1 -> dout_compress/43(in43)
  del44/1 -> dout_compress/44(in44)
  del45/1 -> dout_compress/45(in45)
  del46/1 -> dout_compress/46(in46)
  del47/1 -> dout_compress/47(in47)
  del48/1 -> dout_compress/48(in48)
  dout_compress/1(bus_out) -> dout/1
